simulink model "ABS_Simul"  (R2022b)
settings: Solver=FixedStepAuto  StartTime=0.0  StopTime=10.0  FixedStep=0.001  RelTol=1e-3
values from neighbouring files (symbols this model uses):
  ABS_ONOFF = 1    [ABS_Simul_Initialize.m]
  Brake_Input_Amplitude = 5e6*2    (= 10000000)    [ABS_Simul_Initialize.m]    (also in Long_Simul_1_Initialize.m = 100; Long_Simul_2_Initialize.m = 7500000; Long_Simul_3_Initialize.m = 7500000)
  Brake_Input_start_time = 8    [ABS_Simul_Initialize.m]    (also in Long_Simul_1_Initialize.m; Long_Simul_2_Initialize.m; Long_Simul_3_Initialize.m)
  lr = 1.8    [ABS_Simul_Initialize.m]    (also in ACC_CTG_Multi_Simul_Initialize.m; ACC_Space_Single_Simul_Initialize.m; ACC_Space_multi_Simul_Initialize.m; CruiseControl_Initialize.m)
  m = 1500    [ABS_Simul_Initialize.m]    (also in ACC_CTG_Multi_Simul_Initialize.m; ACC_Space_Single_Simul_Initialize.m; ACC_Space_multi_Simul_Initialize.m; CruiseControl_Initialize.m)
  Slip_thres = 0.13    [ABS_Simul_Initialize.m]
  Throttle_Input_Amplitude = 30    [ABS_Simul_Initialize.m]    (also in Long_Simul_1_Initialize.m; Long_Simul_2_Initialize.m; Long_Simul_3_Initialize.m)
  Throttle_Input_period = 4    [ABS_Simul_Initialize.m]    (also in Long_Simul_1_Initialize.m; Long_Simul_2_Initialize.m; Long_Simul_3_Initialize.m)
libraries: autolibshared x2, autolibsharedmappedengines x1
(part 2 of 2)

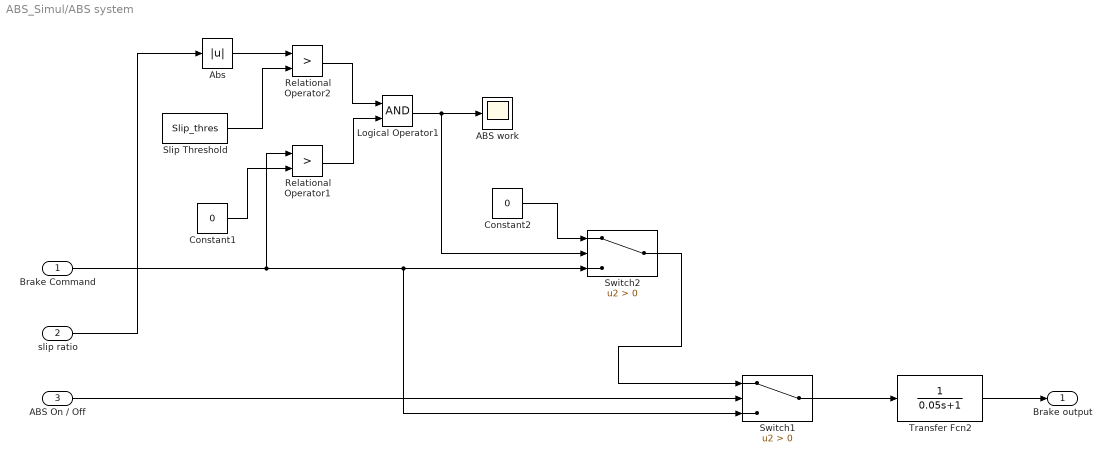
== system ABS_Simul/ABS system ==
  Brake Command : Inport
  slip ratio : Inport  Port=2
  ABS On / Off : Inport  Port=3
  ABS work : Scope
  Abs : Abs  SaturateOnIntegerOverflow=off
  Constant1 : Constant  Value=0
  Constant2 : Constant  Value=0
  Logical Operator1 : Logic  AllPortsSameDT=off  OutDataTypeStr=boolean
  Relational Operator1 : RelationalOperator  Operator=>  OutDataTypeStr=boolean  RndMeth=Simplest  InputSameDT=off
  Relational Operator2 : RelationalOperator  Operator=>  OutDataTypeStr=boolean  RndMeth=Simplest  InputSameDT=off
  Slip Threshold : Constant  Value=Slip_thres
  Switch1 : Switch  Criteria=u2 > Threshold  SaturateOnIntegerOverflow=off  InputSameDT=off
  Switch2 : Switch  Criteria=u2 > Threshold  SaturateOnIntegerOverflow=off  InputSameDT=off
  Transfer Fcn2 : TransferFcn  Denominator=[0.05 1]
  Brake output : Outport
  wires:
  Logical Operator1/1 -> Switch2/2, ABS work/1
  Constant2/1 -> Switch2/1
  Slip Threshold/1 -> Relational Operator2/2
  Constant1/1 -> Relational Operator1/2
  Brake Command/1 -> Switch1/3, Switch2/3, Relational Operator1/1
  Relational Operator1/1 -> Logical Operator1/2
  Relational Operator2/1 -> Logical Operator1/1
  Abs/1 -> Relational Operator2/1
  Transfer Fcn2/1 -> Brake output/1
  slip ratio/1 -> Abs/1
  ABS On / Off/1 -> Switch1/2
  Switch2/1 -> Switch1/1
  Switch1/1 -> Transfer Fcn2/1
